simulink model "TestMotors"  (R2018b)
settings: Solver=VariableStepAuto  StartTime=0.0  StopTime=Simulation.T_END  MaxStep=Simulation.TS_MAX  RelTol=1e-3
undefined symbols (not defined in the file): pwmIn
settings Model: Creator=jeremie  LastModifiedBy=jban039
settings DataIOCC: ReturnWorkspaceOutputs=on
settings SFSimCC: SimUseLocalCustomCode=off
settings RTWCC: RTWUseLocalCustomCode=off
settings CodeAppCC: StateflowObjectComments=on

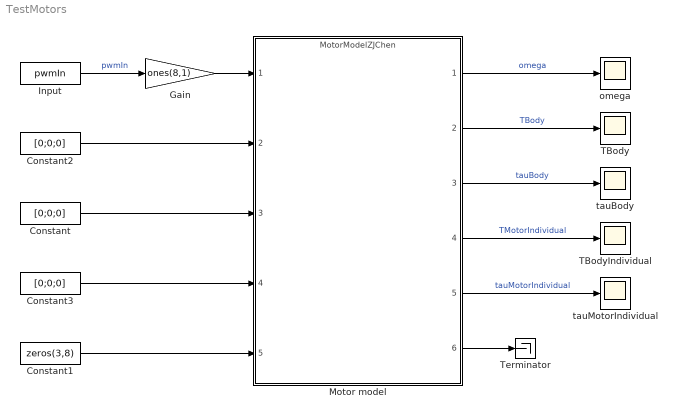
== system TestMotors ==
  Constant : Constant  Value=[0;0;0]
  Constant1 : Constant  Value=zeros(3,8)
  Constant2 : Constant  Value=[0;0;0]
  Constant3 : Constant  Value=[0;0;0]
  Gain : Gain  Gain=ones(8,1)
  Input : Constant  Value=pwmIn
  Motor model : ModelReference  ModelNameDialog=MotorModelZJChen  SimulationMode=Normal  ModelReferenceVersion=1.448
  TBody : Scope
  TBodyIndividual : Scope
  Terminator : Terminator
  omega : Scope
  tauBody : Scope
  tauMotorIndividual : Scope
  wires:
  Constant/1 -> Motor model/3
  Constant1/1 -> Motor model/5
  Constant2/1 -> Motor model/2
  Motor model/6 -> Terminator/1
  Motor model/5 -> tauMotorIndividual/1  "tauMotorIndividual"
  Motor model/4 -> TBodyIndividual/1  "TMotorIndividual"
  Gain/1 -> Motor model/1
  Input/1 -> Gain/1  "pwmIn"
  Motor model/1 -> omega/1  "omega"
  Motor model/2 -> TBody/1  "TBody"
  Motor model/3 -> tauBody/1  "tauBody"
  Constant3/1 -> Motor model/4
